simulink model "lab07"  (R2022b)
settings: Solver=ode45  StartTime=0.0  StopTime=10  FixedStep=0.01  RelTol=1e-3
settings Model: Creator=Lab Admin  LastModifiedBy=Wasif
settings DataIOCC: ReturnWorkspaceOutputs=off
settings DebuggingCC: UnconnectedInputMsg=warning  UnconnectedOutputMsg=warning  UnconnectedLineMsg=warning
settings ModelReferenceCC: EnableRefExpFcnMdlSchedulingChecks=on
settings RTWCC: DLArmComputeVersion=19.05

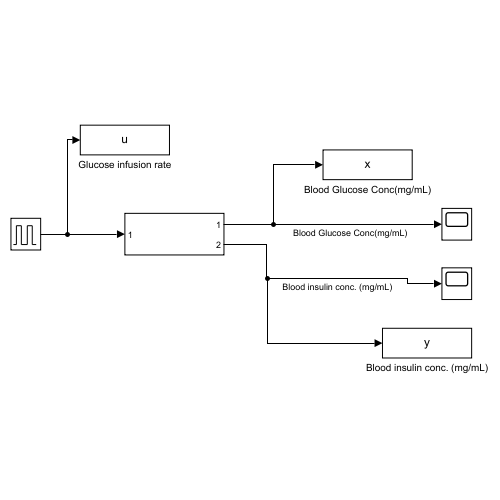
[thumbnail: Simulink's stored preview of the top-level diagram]
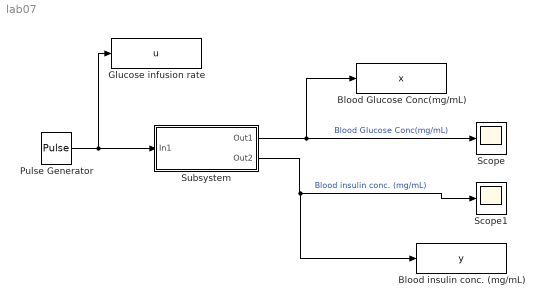
== system lab07 ==
  Blood Glucose Conc(mg/mL) : ToWorkspace  VariableName=x  SampleTime=-1
  Blood insulin conc. (mg/mL) : ToWorkspace  VariableName=y  SampleTime=-1
  Glucose infusion rate : ToWorkspace  VariableName=u  SampleTime=-1
  Pulse Generator : DiscretePulseGenerator  PulseType=Time based  Amplitude=100000  Period=5  PulseWidth=5  PhaseDelay=0.5
  Scope : Scope
  Scope1 : Scope
  Subsystem : Subsystem
  wires:
  Pulse Generator/1 -> Glucose infusion rate/1, Subsystem/1(In1)
  Subsystem/1(Out1) -> Blood Glucose Conc(mg/mL)/1, Scope/1  "Blood Glucose Conc(mg/mL)"
  Subsystem/2(Out2) -> Blood insulin conc. (mg/mL)/1, Scope1/1  "Blood insulin conc. (mg/mL)"

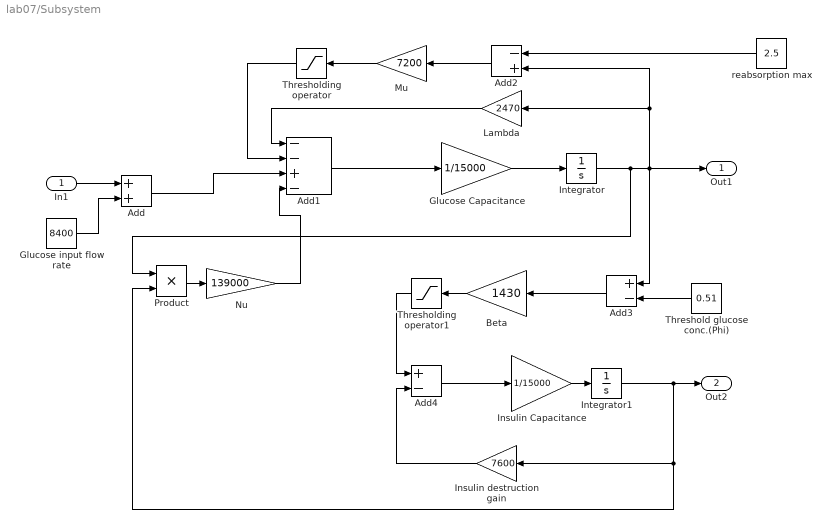
== system lab07/Subsystem ==
  In1 : Inport
  Add : Sum
  Add1 : Sum  Inputs=--+-
  Add2 : Sum  Inputs=-+
  Add3 : Sum  Inputs=+-
  Add4 : Sum  Inputs=+-
  Beta : Gain  Gain=1430
  Glucose Capacitance : Gain  Gain=1/15000
  Glucose input flow rate : Constant  Value=8400
  Insulin Capacitance : Gain  Gain=1/15000
  Insulin destruction gain : Gain  Gain=7600
  Integrator : Integrator  InitialCondition=0.81
  Integrator1 : Integrator  InitialCondition=0.055
  Lambda : Gain  Gain=2470
  Mu : Gain  Gain=7200
  Nu : Gain  Gain=139000
  Product : Product
  Threshold glucose conc.(Phi) : Constant  Value=0.51
  Thresholding operator : Saturate  UpperLimit=10000  LowerLimit=0
  Thresholding operator1 : Saturate  UpperLimit=10000  LowerLimit=0
  reabsorption max : Constant  Value=2.5
  Out1 : Outport
  Out2 : Outport  Port=2
  wires:
  In1/1 -> Add/1
  Glucose input flow rate/1 -> Add/2
  Add/1 -> Add1/3
  Add1/1 -> Glucose Capacitance/1
  Glucose Capacitance/1 -> Integrator/1
  Integrator/1 -> Product/1, Out1/1, Add2/2, Lambda/1, Add3/1
  Lambda/1 -> Add1/1
  reabsorption max/1 -> Add2/1
  Add2/1 -> Mu/1
  Mu/1 -> Thresholding operator/1
  Thresholding operator/1 -> Add1/2
  Threshold glucose conc.(Phi)/1 -> Add3/2
  Add3/1 -> Beta/1
  Beta/1 -> Thresholding operator1/1
  Thresholding operator1/1 -> Add4/1
  Add4/1 -> Insulin Capacitance/1
  Insulin Capacitance/1 -> Integrator1/1
  Integrator1/1 -> Insulin destruction gain/1, Product/2, Out2/1
  Insulin destruction gain/1 -> Add4/2
  Nu/1 -> Add1/4
  Product/1 -> Nu/1
